simulink model "Unfolded and redesigned recursive architecture"  (R2015b)
settings: Solver=VariableStepAuto  StartTime=0.0  StopTime=10.0  RelTol=1e-3
libraries: shlslibv1 x24
settings Model: synDspstartup=None  Creator=sjparekh  LastModifiedBy=sjparekh
settings DebuggingCC: InheritedTsInSrcMsg=none

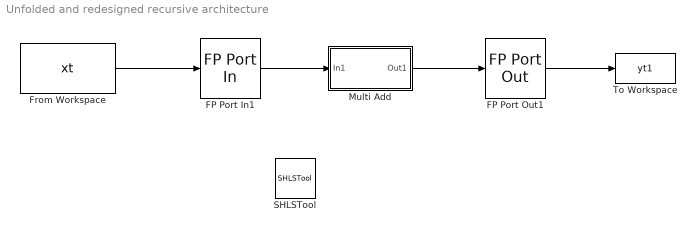
== system Unfolded and redesigned recursive architecture ==
  FP Port In1 : shlslibv1/Floating Point/FP Port In  synBlockType=custom  synLatency=1  syn_exp_wl=8  syn_frac_wl=20  syn_out_st=1/258.4e6  syn_capture=on  syn_register=on  syn_opt_ports=off
  FP Port Out1 : shlslibv1/Floating Point/FP Port Out  synBlockType=custom  synLatency=1  syn_exp_wl=8  syn_frac_wl=20  syn_capture=on  syn_register=on
  From Workspace : FromWorkspace  VariableName=xt  SampleTime=1/258.4e6  OutputAfterFinalValue=Holding final value
  Multi Add : Subsystem
  SHLSTool : shlslibv1/SHLSTool  synBlockType=tool  syn_dsp_mode=FPGA
  To Workspace : ToWorkspace  VariableName=yt1  SaveFormat=Structure With Time  SampleTime=1/258.4e6
  wires:
  From Workspace/1 -> FP Port In1/1
  FP Port In1/1 -> Multi Add/1(In1)
  Multi Add/1(Out1) -> FP Port Out1/1
  FP Port Out1/1 -> To Workspace/1

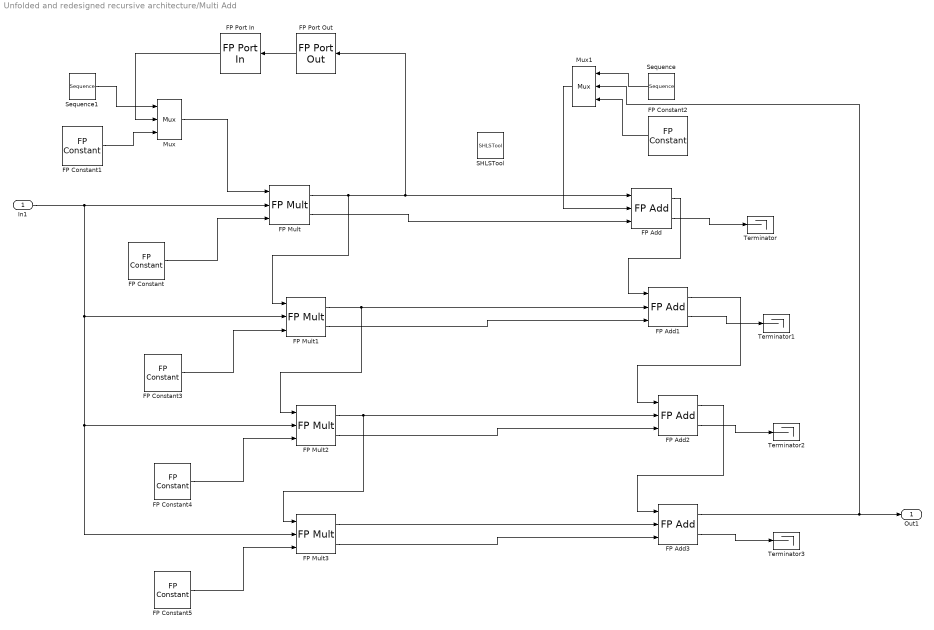
== system Unfolded and redesigned recursive architecture/Multi Add ==
  In1 : Inport
  FP Add{,1..3} (4 alike) : shlslibv1/Floating Point/FP Add  syn_exp_wl=8  syn_frac_wl=20  syn_opt_ports=off  syn_add_opr=add  synBlockType=custom  synLatency=9
  FP Constant{,1,3..5} (5 alike) : shlslibv1/Floating Point/FP Constant  syn_constant_val=1  syn_exp_wl=8  syn_frac_wl=20  syn_cst_st=-1  synBlockType=custom  synLatency=0
  FP Constant2 : shlslibv1/Floating Point/FP Constant  syn_constant_val=8  syn_exp_wl=20  syn_frac_wl=23  syn_cst_st=-1  synBlockType=custom  synLatency=0
  FP Mult{,1..3} (4 alike) : shlslibv1/Floating Point/FP Mult  syn_exp_wl=8  syn_frac_wl=20  syn_opt_ports=off  synBlockType=custom  synLatency=9  syn_opt_tar=Default  syn_fracmult_pipe=7
  FP Port In : shlslibv1/Floating Point/FP Port In  synBlockType=custom  synLatency=1  syn_exp_wl=8  syn_frac_wl=20  syn_out_st=-1  syn_capture=on  syn_register=on  syn_opt_ports=off
  FP Port Out : shlslibv1/Floating Point/FP Port Out  synBlockType=custom  synLatency=1  syn_exp_wl=8  syn_frac_wl=20  syn_capture=on  syn_register=on
  Mux : shlslibv1/Signal Operations/Mux  syn_in_nb=2  syn_out_f=Full Precision  syn_out_wl=16  syn_out_fl=8  syn_out_dt=signed  syn_en_se=off  synBlockType=primitive  synLatency=0  synBlockId=16
  Mux1 : shlslibv1/Signal Operations/Mux  syn_in_nb=2  syn_out_f=Full Precision  syn_out_wl=16  syn_out_fl=8  syn_out_dt=signed  syn_en_se=off  synBlockType=primitive  synLatency=0  synBlockId=16
  SHLSTool : shlslibv1/SHLSTool  synBlockType=tool  syn_dsp_mode=FPGA
  Sequence : shlslibv1/Sources/Sequence  syn_seq_vec=[1 1 1 1 1 1 1 1 zeros(1,1000)]  syn_seq_wl=16  syn_seq_fl=8  syn_seq_dt=signed  syn_rst_port=off  syn_en_port=off  syn_seq_st=-1  synBlockType=custom  synLatency=1
  Sequence1 : shlslibv1/Sources/Sequence  syn_seq_vec=[1 zeros(1,899)]  syn_seq_wl=16  syn_seq_fl=8  syn_seq_dt=signed  syn_rst_port=off  syn_en_port=off  syn_seq_st=-1  synBlockType=custom  synLatency=1
  Terminator{,1..3} (4 alike) : Terminator
  Out1 : Outport
  wires:
  FP Constant/1 -> FP Mult/3
  In1/1 -> FP Mult3/2, FP Mult2/2, FP Mult1/2, FP Mult/2
  Mux/1 -> FP Mult/1
  FP Constant1/1 -> Mux/3
  FP Mult/2 -> FP Add/3
  FP Mult/1 -> FP Mult1/1, FP Add/1, FP Port Out/1
  FP Port Out/1 -> FP Port In/1
  FP Port In/1 -> Mux/2
  FP Constant2/1 -> Mux1/3
  FP Add/2 -> Terminator/1
  FP Constant3/1 -> FP Mult1/3
  FP Constant4/1 -> FP Mult2/3
  FP Add1/2 -> Terminator1/1
  Sequence1/1 -> Mux/1
  Sequence/1 -> Mux1/1
  FP Add/1 -> FP Add1/1
  FP Mult1/1 -> FP Mult2/1, FP Add1/2
  FP Mult1/2 -> FP Add1/3
  FP Constant5/1 -> FP Mult3/3
  FP Add2/2 -> Terminator2/1
  FP Add1/1 -> FP Add2/1
  FP Mult2/1 -> FP Mult3/1, FP Add2/2
  FP Mult2/2 -> FP Add2/3
  FP Add3/2 -> Terminator3/1
  FP Add2/1 -> FP Add3/1
  FP Mult3/1 -> FP Add3/2
  FP Mult3/2 -> FP Add3/3
  FP Add3/1 -> Mux1/2, Out1/1
  Mux1/1 -> FP Add/2
